simulink model "controller_velocity_MPC"  (R2021a)
settings: Solver=FixedStepAuto  StartTime=0.0  StopTime=10  RelTol=1e-3
undefined symbols (not defined in the file): max_tilt, payload_angle_ref, sim_freq, thr_max, thr_min, Ts_mpc, u_bar
libraries: mpclib x1
settings Model: Creator=francois  LastModifiedBy=esl
settings SolverCC: AlgebraicLoopSolver=TrustRegion
settings DataIOCC: SaveOutput=off  SaveTime=off
settings DebuggingCC: SFMachineParentedDataDiag=warning
settings ModelReferenceCC: ModelReferenceNumInstancesAllowed=Single

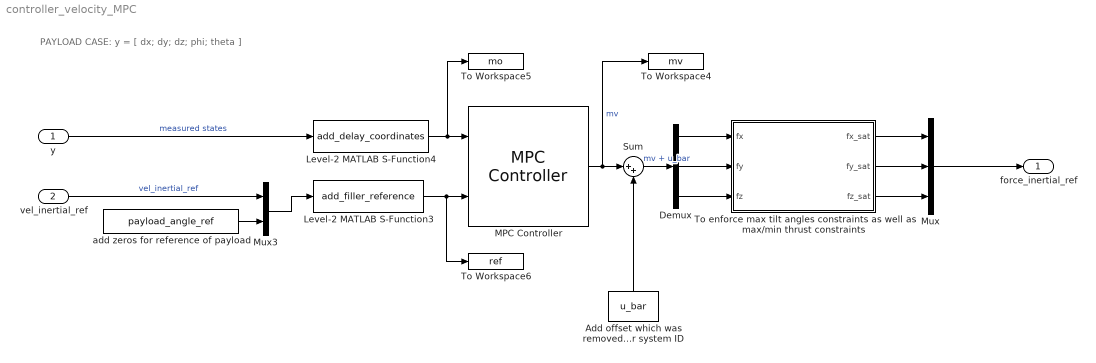
== system controller_velocity_MPC ==
  note: PAYLOAD CASE: y = [ dx; dy; dz; phi; theta ]
  y : Inport  OutDataTypeStr=double  PortDimensions=5  SampleTime=[0.002,0]
  vel_inertial_ref : Inport  Port=2  OutDataTypeStr=double  PortDimensions=3  SampleTime=0
  Add offset which was removed for system ID : Constant  Value=u_bar
  Demux : Demux  Outputs=3
  Level-2 MATLAB S-Function3 : M-S-Function  FunctionName=add_filler_reference  Parameters=ny, q, Ts_mpc
  Level-2 MATLAB S-Function4 : M-S-Function  FunctionName=add_delay_coordinates  Parameters=y_ext_0, q, Ts_mpc, ny
  MPC Controller : mpclib/MPC Controller  SCDEnableBlockLinearizationSpecification=on  mpcobj=mpc_vel  is_multiple=0  enable_value=0  return_u0=off  updateMPCinCallerWorkspace=on  md_inport=off  mv_inport=off  uref_inport=off  return_cost=off  return_mvseq=off  return_qpstatus=off  return_xseq=off  return_state=off  return_ovseq=off  state_inport=off  umin_inport=off  umax_inport=off  ymin_inport=off  ymax_inport=off  cc_inport=off  ywt_inport=off  uwt_inport=off  duwt_inport=off  rhoeps_inport=off  pm_inport=off  MaximumP=10  HorizonChoice=FixedHorizon  n_ts=0.03  n_p=200  n_mv=3  n_md=0  n_ud=0  n_mo=60  n_uo=0  BlockDataType=double  SampleTimeInherited=off  switch_inport=off
  Mux : Mux  Inputs=3
  Mux3 : Mux  Inputs=2
  Sum : Sum  Inputs=|++
  To Workspace4 : ToWorkspace  VariableName=mv  SaveFormat=Timeseries  SampleTime=Ts_mpc
  To Workspace5 : ToWorkspace  VariableName=mo  SaveFormat=Timeseries  SampleTime=Ts_mpc
  To Workspace6 : ToWorkspace  VariableName=ref  SaveFormat=Timeseries  SampleTime=Ts_mpc
  To enforce max tilt angles constraints as well as max/min thrust constraints : MATLAB Function  TreatAsAtomicUnit=on  SystemSampleTime=1/sim_freq
  add zeros for reference of payload : Constant  Value=payload_angle_ref
  force_inertial_ref : Outport  OutDataTypeStr=double  PortDimensions=3  SampleTime=[0.002,0]
  wires:
  Level-2 MATLAB S-Function3/1 -> MPC Controller/2, To Workspace6/1
  Level-2 MATLAB S-Function4/1 -> MPC Controller/1, To Workspace5/1
  To enforce max tilt angles constraints as well as max/min thrust constraints/3(fz_sat) -> Mux/3
  To enforce max tilt angles constraints as well as max/min thrust constraints/1(fx_sat) -> Mux/1
  To enforce max tilt angles constraints as well as max/min thrust constraints/2(fy_sat) -> Mux/2
  Demux/2 -> To enforce max tilt angles constraints as well as max/min thrust constraints/2(fy)
  Demux/3 -> To enforce max tilt angles constraints as well as max/min thrust constraints/3(fz)
  Demux/1 -> To enforce max tilt angles constraints as well as max/min thrust constraints/1(fx)
  Mux/1 -> force_inertial_ref/1
  MPC Controller/1 -> Sum/1, To Workspace4/1  "mv"
  Sum/1 -> Demux/1  "mv + u_bar"
  Add offset which was removed for system ID/1 -> Sum/2
  y/1 -> Level-2 MATLAB S-Function4/1  "measured states"
  add zeros for reference of payload/1 -> Mux3/2
  vel_inertial_ref/1 -> Mux3/1  "vel_inertial_ref"
  Mux3/1 -> Level-2 MATLAB S-Function3/1

== matlab function controller_velocity_MPC/To enforce max tilt angles constraints as well as max//min thrust constraints ==
  data: fx input; fx_sat output; fy input; fz input; fy_sat output; max_tilt parameter; thr_max parameter; fz_sat output; thr_min parameter
function [fx_sat, fy_sat, fz_sat] = constrain_max_tilt(fx, fy, fz, max_tilt, thr_max, thr_min)
    % First constrain fz.
    if fz > -thr_min
        fz_sat = -thr_min;
    elseif fz < -thr_max
        fz_sat = -thr_max;
    else
        fz_sat = fz;
    end
    
    % Constrain fx and fy
    thrust_max_NE_tilt = abs(fz_sat) * tan(max_tilt * pi/180);
    thrust_max_NE = sqrt(thr_max*thr_max - fz_sat*fz_sat);
    thrust_max_NE = min(thrust_max_NE_tilt, thrust_max_NE);
    
    fx_sat = fx;
    fy_sat = fy;

%     if dot([fx, fy], [fx, fy]) > thrust_max_NE*thrust_max_NE
%         mag = norm([fx, fy]);
    mag = norm([fx, fy]); %myne
    if mag > thrust_max_NE% myne
        fx_sat = fx / mag * thrust_max_NE;
        fy_sat = fy / mag * thrust_max_NE;
    end
end
